simulink model "TurnLightAct_backup"  (R2023a)
settings: Solver=FixedStepDiscrete  StartTime=0.0  StopTime=10.0  FixedStep=0.01  RelTol=1e-3
libraries: TurnLightMode_Control x4
settings Model: Creator=19856  LastModifiedBy=19856
settings DataIOCC: SaveFormat=StructureWithTime
settings OptimizationCC: DefaultParameterBehavior=Inlined  EnhancedBackFolding=on  PassReuseOutputArgsAs=Individual arguments  ZeroExternalMemoryAtStartup=off  ZeroInternalMemoryAtStartup=off  OptimizeBlockOrder=speed  DifferentSizesBufferReuse=on  OptimizationCustomize=off  EfficientTunableParamExpr=on
settings DebuggingCC: ParameterTunabilityLossMsg=error
settings ModelReferenceCC: ModelReferenceNumInstancesAllowed=Single
settings SFSimCC: MATLABDynamicMemAlloc=off
settings RTWCC: Description=AUTOSAR  SystemTargetFile=autosar.tlc  GenCodeOnly=on  TemplateMakefile=ert_default_tmf
settings CodeAppCC: ForceParamTrailComments=on  IgnoreCustomStorageClasses=off  OperatorAnnotations=on  SimulinkDataObjDesc=on  SFDataObjDesc=on  InsertBlockDesc=on
settings STFCustomTargetCC: MultiwordLength=256  ParMdlRefBuildCompliant=on  CompOptLevelCompliant=on  ConcurrentExecutionCompliant=off  IncludeMdlTerminateFcn=off  CombineOutputUpdateFcns=on  SuppressErrorStatus=on  ERTCustomFileBanners=on  SupportNonFinite=off  SupportComplex=off  SupportContinuousTime=off  SupportNonInlinedSFcns=off  RemoveResetFunc=on  MATLABClassNameForMDSCustomization=Simulink.SoftwareTarget.ERTCustomization  AutosarCompliant=on  GRTInterface=off  LookupTableObjectStructAxisOrder=2,1,3,4,...  LUTObjectStructOrderEvenSpacing=Size,Table,Breakpoints  SystemTargetFile=autosar.tlc
settings ERTTargetCC: TargetLangStandard=C99 (ISO)  ConcurrentExecutionCompliant=off  IncludeMdlTerminateFcn=off  SuppressErrorStatus=on  SupportNonFinite=off  SupportComplex=off  ModelStepFunctionPrototypeControlCompliant=off  CPPClassGenCompliant=off  AutosarCompliant=on  LookupTableObjectStructAxisOrder=2,1,3,4,...  LUTObjectStructOrderEvenSpacing=Size,Table,Breakpoints  InlinedParameterPlacement=NonHierarchical  ERTCustomFileTemplate=example_file_process.tlc

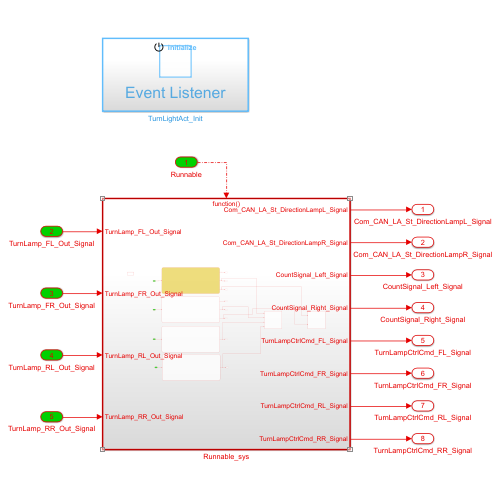
[thumbnail: Simulink's stored preview of the top-level diagram]
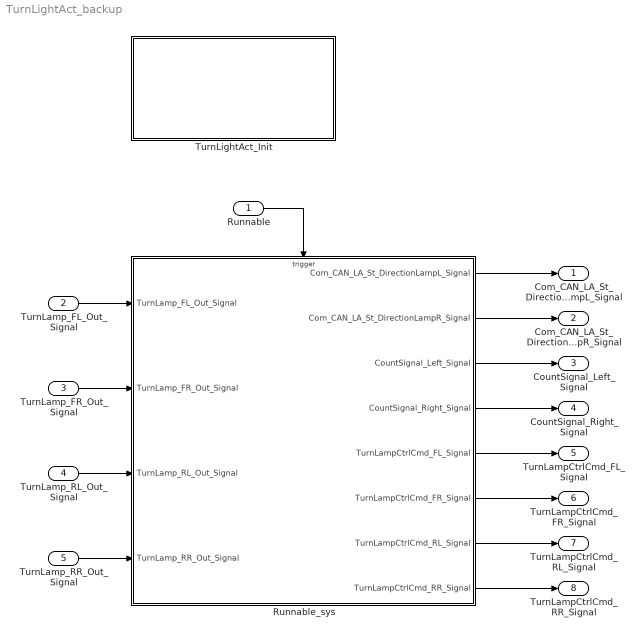
== system TurnLightAct_backup ==
  Runnable : Inport  SampleTime=0.01  OutputFunctionCall=on
  TurnLamp_FL_Out_Signal : Inport  Port=2  OutDataTypeStr=uint8  PortDimensions=1
  TurnLamp_FR_Out_Signal : Inport  Port=3  OutDataTypeStr=uint8  PortDimensions=1
  TurnLamp_RL_Out_Signal : Inport  Port=4  OutDataTypeStr=uint8  PortDimensions=1
  TurnLamp_RR_Out_Signal : Inport  Port=5  OutDataTypeStr=uint8  PortDimensions=1
  Runnable_sys : Subsystem
  TurnLightAct_Init : Subsystem
  Com_CAN_LA_St_DirectionLampL_Signal : Outport  OutDataTypeStr=uint8  PortDimensions=1
  Com_CAN_LA_St_DirectionLampR_Signal : Outport  Port=2  OutDataTypeStr=uint8  PortDimensions=1
  CountSignal_Left_Signal : Outport  Port=3  OutDataTypeStr=uint8  PortDimensions=1
  CountSignal_Right_Signal : Outport  Port=4  OutDataTypeStr=uint8  PortDimensions=1
  TurnLampCtrlCmd_FL_Signal : Outport  Port=5  OutDataTypeStr=uint8  PortDimensions=1
  TurnLampCtrlCmd_FR_Signal : Outport  Port=6  OutDataTypeStr=uint8  PortDimensions=1
  TurnLampCtrlCmd_RL_Signal : Outport  Port=7  OutDataTypeStr=uint8  PortDimensions=1
  TurnLampCtrlCmd_RR_Signal : Outport  Port=8  OutDataTypeStr=uint8  PortDimensions=1
  wires:
  TurnLamp_FL_Out_Signal/1 -> Runnable_sys/1(TurnLamp_FL_Out_Signal)
  TurnLamp_FR_Out_Signal/1 -> Runnable_sys/2(TurnLamp_FR_Out_Signal)
  TurnLamp_RL_Out_Signal/1 -> Runnable_sys/3(TurnLamp_RL_Out_Signal)
  TurnLamp_RR_Out_Signal/1 -> Runnable_sys/4(TurnLamp_RR_Out_Signal)
  Runnable_sys/1(Com_CAN_LA_St_DirectionLampL_Signal) -> Com_CAN_LA_St_DirectionLampL_Signal/1
  Runnable_sys/2(Com_CAN_LA_St_DirectionLampR_Signal) -> Com_CAN_LA_St_DirectionLampR_Signal/1
  Runnable_sys/3(CountSignal_Left_Signal) -> CountSignal_Left_Signal/1
  Runnable_sys/4(CountSignal_Right_Signal) -> CountSignal_Right_Signal/1
  Runnable_sys/5(TurnLampCtrlCmd_FL_Signal) -> TurnLampCtrlCmd_FL_Signal/1
  Runnable_sys/6(TurnLampCtrlCmd_FR_Signal) -> TurnLampCtrlCmd_FR_Signal/1
  Runnable_sys/7(TurnLampCtrlCmd_RL_Signal) -> TurnLampCtrlCmd_RL_Signal/1
  Runnable_sys/8(TurnLampCtrlCmd_RR_Signal) -> TurnLampCtrlCmd_RR_Signal/1
  Runnable/1 -> Runnable_sys/Trigger

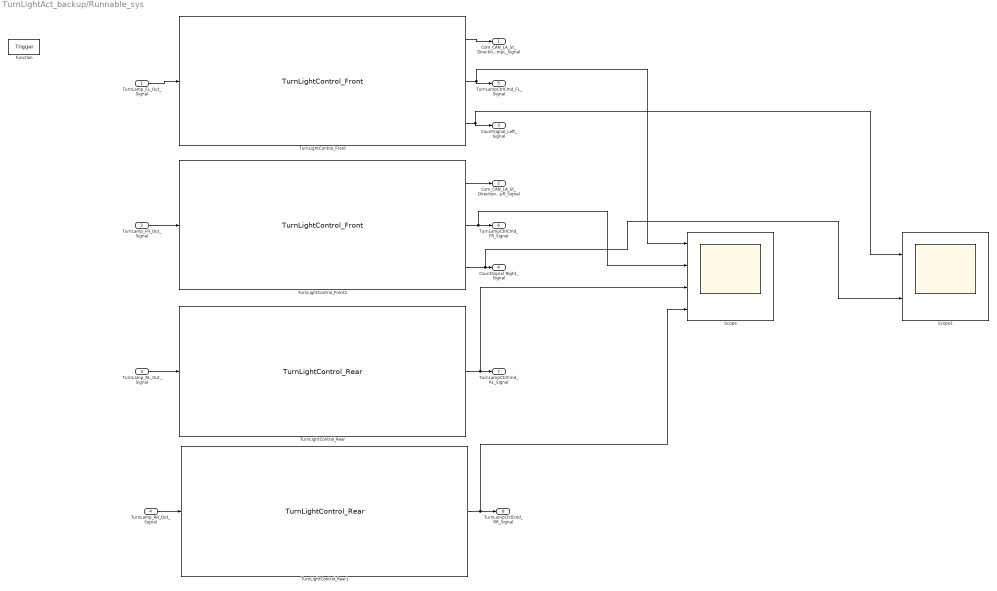
== system TurnLightAct_backup/Runnable_sys ==
  TurnLamp_FL_Out_Signal : Inport
  TurnLamp_FR_Out_Signal : Inport  Port=2
  TurnLamp_RL_Out_Signal : Inport  Port=3
  TurnLamp_RR_Out_Signal : Inport  Port=4
  function : TriggerPort  TriggerType=function-call  VariantControl=(inherit)  SampleTimeType=periodic  SampleTime=-1
  Scope : Scope  NumInputPorts=4
  Scope1 : Scope  NumInputPorts=2
  TurnLightControl_Front : TurnLightMode_Control/TurnLightControl_Front  SystemSampleTime=-1  VariantActivationTime=update diagram  Latency=0  AutoFrameSizeCalculation=off
      settings: SourceProductName=My Library_TurnLightLightMode_Control
  TurnLightControl_Front1 : TurnLightMode_Control/TurnLightControl_Front  SystemSampleTime=-1  VariantActivationTime=update diagram  Latency=0  AutoFrameSizeCalculation=off
      settings: SourceProductName=My Library_TurnLightLightMode_Control
  TurnLightControl_Rear : TurnLightMode_Control/TurnLightControl_Rear  SystemSampleTime=-1  VariantActivationTime=update diagram  Latency=0  AutoFrameSizeCalculation=off
      settings: SourceProductName=My Library_TurnLightLightMode_Control
  TurnLightControl_Rear1 : TurnLightMode_Control/TurnLightControl_Rear  SystemSampleTime=-1  VariantActivationTime=update diagram  Latency=0  AutoFrameSizeCalculation=off
      settings: SourceProductName=My Library_TurnLightLightMode_Control
  Com_CAN_LA_St_DirectionLampL_Signal : Outport
      settings: EnsureOutportIsVirtual=on
  Com_CAN_LA_St_DirectionLampR_Signal : Outport  Port=2
      settings: EnsureOutportIsVirtual=on
  CountSignal_Left_Signal : Outport  Port=3
      settings: EnsureOutportIsVirtual=on
  CountSignal_Right_Signal : Outport  Port=4
      settings: EnsureOutportIsVirtual=on
  TurnLampCtrlCmd_FL_Signal : Outport  Port=5
      settings: EnsureOutportIsVirtual=on
  TurnLampCtrlCmd_FR_Signal : Outport  Port=6
      settings: EnsureOutportIsVirtual=on
  TurnLampCtrlCmd_RL_Signal : Outport  Port=7
      settings: EnsureOutportIsVirtual=on
  TurnLampCtrlCmd_RR_Signal : Outport  Port=8
      settings: EnsureOutportIsVirtual=on
  wires:
  TurnLamp_FL_Out_Signal/1 -> TurnLightControl_Front/1
  TurnLamp_FR_Out_Signal/1 -> TurnLightControl_Front1/1
  TurnLamp_RL_Out_Signal/1 -> TurnLightControl_Rear/1
  TurnLamp_RR_Out_Signal/1 -> TurnLightControl_Rear1/1
  TurnLightControl_Front/1 -> Com_CAN_LA_St_DirectionLampL_Signal/1
  TurnLightControl_Front/3 -> CountSignal_Left_Signal/1, Scope1/1
  TurnLightControl_Front/2 -> TurnLampCtrlCmd_FL_Signal/1, Scope/1
  TurnLightControl_Rear/1 -> Scope/3, TurnLampCtrlCmd_RL_Signal/1
  TurnLightControl_Rear1/1 -> Scope/4, TurnLampCtrlCmd_RR_Signal/1
  TurnLightControl_Front1/2 -> Scope/2, TurnLampCtrlCmd_FR_Signal/1
  TurnLightControl_Front1/3 -> Scope1/2, CountSignal_Right_Signal/1
  TurnLightControl_Front1/1 -> Com_CAN_LA_St_DirectionLampR_Signal/1

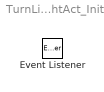
== system TurnLightAct_backup/TurnLightAct_Init ==
  Event Listener : EventListener  EventName=reset
